simulink model "UnitTest_relay_model"  (Simulink 8.1)
settings: Solver=ode1  StartTime=0.0  StopTime=inf  FixedStep=Ts  MaxStep=1e-3  RelTol=1e-3
model workspace (MAT data in the model file):
  op_snapshot1 : opcond.OperatingPoint (value not decoded)
PostLoadFcn:
  | UnitTest_relay_model_init;
InitFcn:
  | UnitTest_relay_model_init;
values from neighbouring files (symbols this model uses):
  relay_par = xlsread('relay_parameters.xlsx')    [relay_settings_init.m]
  Ts = 100E-6    (= 0.0001)    [UnitTest_relay_model_init.m]
undefined symbols (not defined in the file or in its folder): cable_spec
libraries: powerlib x2, artemis x1, rtlab x1, breaker_lib x1, Load_lib x1, relay_modbus_lib x1, rtio_generic_modbus x1, cables_lib x1, transformer_lib x1
settings Model: ARTEMISmethode_block_infos=$$__separator__$$UnitTest_relay_model/ARTEMIS Guide$$__separator__$$  Creator=RE25624  LastModifiedBy=re25624  BufferReuse=off
settings SolverCC: ZeroCrossAlgorithm=Adaptive
settings DataIOCC: ExternalInput=getinputstruct(op_snapshot1)  InitialState=getstatestruct(op_snapshot1)  LimitDataPoints=off  MaxDataPoints=90060  SignalLoggingSaveFormat=Dataset  SaveOutput=off  SignalLogging=off  DSMLogging=off  SaveTime=off  OutputSaveName=result
settings OptimizationCC: BlockReduction=off  OptimizeBlockIOStorage=off  BufferReuse=off  ExpressionFolding=off  LocalBlockOutputs=off
settings DebuggingCC: MaxConsecutiveZCsMsg=warning  IgnoredZcDiagnostic=none  SolverPrmCheckMsg=none  MultiTaskRateTransMsg=warning  FcnCallInpInsideContextMsg=EnableAllAsWarning  FrameProcessingCompatibilityMsg=error  ModelReferenceExtraNoncontSigs=warning  StrictBusMsg=None
settings ModelReferenceCC: UpdateModelReferenceTargets=IfOutOfDate
settings SFSimCC: SFSimEcho=off
settings GRTTargetCC: CodeReplacementLibrary=C89/C90 (ANSI)

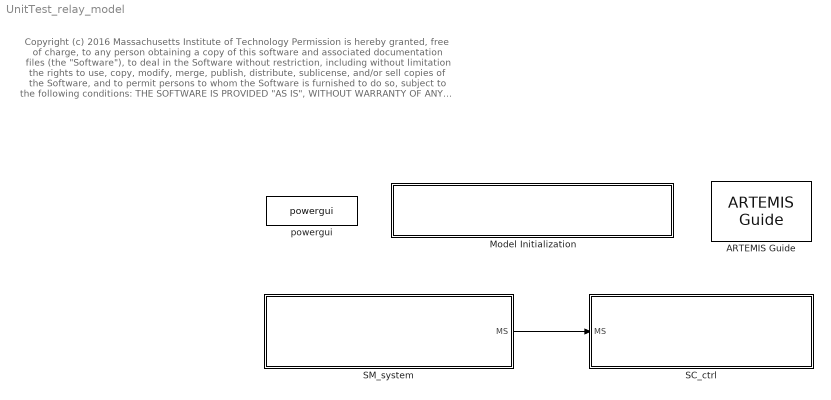
== system UnitTest_relay_model ==
  note: Copyright (c) 2016 Massachusetts Institute of Technology
      | Permission is hereby granted, free of charge, to any person obtaining a copy of this software and associated documentation files (the "Software"), to deal
      | in the Software without restriction, including without limitation the rights to use, copy, modify, merge, publish, distribute, sublicense, and/or sell copies of the
      | Software, and to permit persons to whom the Software is furnished to do so, subject to the following conditions:
      |
      | THE SOFTWARE IS PROVIDED "AS IS", WITHOUT WARRANTY OF ANY KIND, EXPRESS OR IMPLIED, INCLUDING BUT NOT LIMITED TO THE
      | WARRANTIES OF MERCHANTABILITY, FITNESS FOR A PARTICULAR PURPOSE AND NONINFRINGEMENT. IN NO EVENT SHALL THE AUTHORS
      | OR COPYRIGHT HOLDERS BE LIABLE FOR ANY CLAIM, DAMAGES OR OTHER LIABILITY, WHETHER IN AN ACTION OF CONTRACT, TORT OR
      | OTHERWISE, ARISING FROM, OUT OF OR IN CONNECTION WITH THE SOFTWARE OR THE USE OR OTHER DEALINGS IN THE SOFTWARE.
  ARTEMIS Guide : artemis/ARTEMIS/ARTEMIS Guide  Tag=FTSSmethode_opal_4hx0r99  Description=5.0_z1  lock=on  Ts=Ts  opt=art5  dyna=off  nb_perm=4  RT_fullcomp=off  ssn=on  ssn_itvc=off  ssn_ivic=off  ssn_ext=off  ssn_solver=Art5 with Backward Euler nodal interface  ssn_impulse=off  ssn_quasimpulse=off  ssn_impulse_loop=2  paraExtinctionThy=off  Thy_Impulse=on  dtc=Off  dtc_opt=normal  ao=on  simtype=off  ct_mac=off  lin_mov=off  lsp=[0.001 2]  spike_skip=Disabled  dtc_extra=1  dtc_sws=normal  dtc_pied=0.5  SPSRulesBlock=SPSRules  tre=on  ctmm=off  LF=off  dpl_type=ARTEMiS DPL  rlc_type=off  custom_type=off  para=on  ssn_ImpulseLoopBlockedStateUpdate=2  ssn_mov_iter_number=5  ssn_switch_iter_number=5
  Model Initialization : Subsystem  AncestorBlock=artemis/Tools /Misc/Model Initialization  mask(Model Functions){InitFcnX=UnitTest_relay_model_init;, prel=off, posl=on, inif=on, strf=off}
      mask prompts: InitFcnX "Initialisation"; prel "Preload Function"; posl "PostLoad Function"; inif "InitFcn"; strf "StartFcn"
      mask init:
      | currentBlock = gcb;
      | root = bdroot(currentBlock);
      | 
      | 
      | if ~strcmp(get_param(root,'BlockDiagramType'),'library')
      |     if prel==1
      |         set_param(root, 'PreLoadFcn', InitFcnX);
      |     else
      |         set_param(root, 'PreLoadFcn', '');
      |     end
      |     if inif==1
      |         set_param(root, 'InitFcn', InitFcnX);
      |     else
      |         set_param(root, 'InitFcn', '');
      |     end
      |     if strf==1
      |         set_param(root, 'StartFcn', InitFcnX);
      |     else
      |         set_param(root, 'StartFcn', '');
      |     end
      |     if posl==1
      |         set_param(root, 'PostLoadFcn', InitFcnX);
      |     else
      |         set_param(root, 'PostLoadFcn', '');
      |     end
      | end
      | 
      | pos = get_param(currentBlock, 'Position');
      | width = pos(3) - pos(1); height = pos(4) - pos(2);
      | txt = [ upper(root) '\n' '- InitFcn. . . . . '  get_param(root, 'InitFcn') ];
      settings: CopyFcn=set_param(gcb,'LinkStatus','inactive')
      mask Display: text(5, height*0.5, txt, 'horizontalAlignment', 'left', 'verticalAlignment', 'middle') ;
  SC_ctrl : Subsystem
  SM_system : Subsystem
  powergui : powerlib/powergui  Priority=2  SimulationMode=Discrete  SolverType=Tustin  SampleTime=Ts  frequency=60  SPID=off  DisableSnubberDevices=off  DisableRonSwitches=off  DisableVfSwitches=off  SwTol=0  Interpol=off  DisplayEquations=off  frequencyindice=0  Pbase=100e6  ErrMax=1e-4  Iterations=50  UnitsV=kV  UnitsW=MW  FunctionMessages=off  echomessages=off  HookPort=off  EnableUseOfTLC=off  x0status=blocks  RestoreLinks=warning  ResistiveCurrentMeasurement=off  Frange=logspace(0,3,50)  Ylog=off  Xlog=off  ShowGrid=off  save=off  variable=ZData  structure=0  ZoomFFT=on  StartTime=0.0  cycles=2  DisplayStyle=off  fundamental=60  FreqAxis=off  MaxFrequency=1000  frequencyindicesteady=1  RmsSteady=1  display=off  Ts=0  methode=off
  wires:
  SM_system/1(MS) -> SC_ctrl/1(MS)

== system UnitTest_relay_model/Model Initialization ==

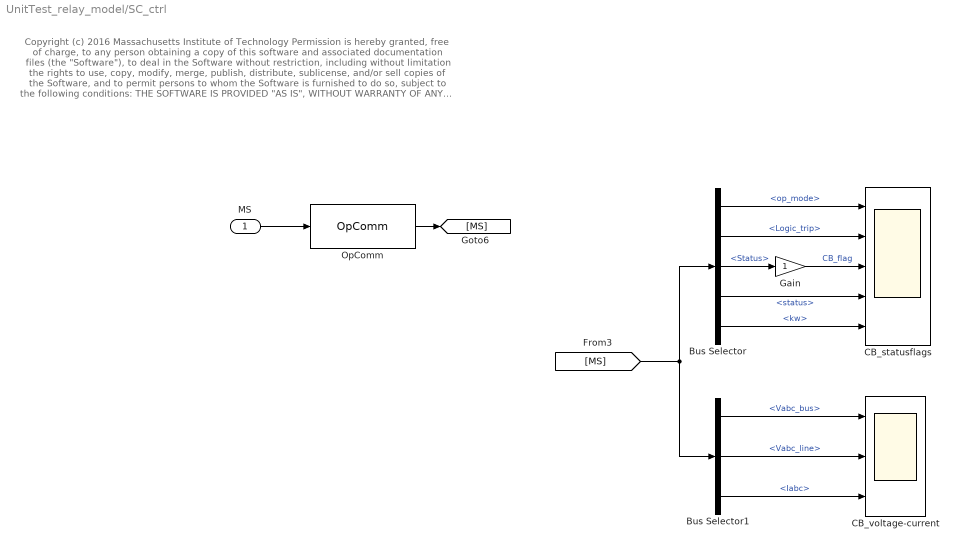
== system UnitTest_relay_model/SC_ctrl ==
  note: Copyright (c) 2016 Massachusetts Institute of Technology
      | Permission is hereby granted, free of charge, to any person obtaining a copy of this software and associated documentation files (the "Software"), to deal
      | in the Software without restriction, including without limitation the rights to use, copy, modify, merge, publish, distribute, sublicense, and/or sell copies of the
      | Software, and to permit persons to whom the Software is furnished to do so, subject to the following conditions:
      |
      | THE SOFTWARE IS PROVIDED "AS IS", WITHOUT WARRANTY OF ANY KIND, EXPRESS OR IMPLIED, INCLUDING BUT NOT LIMITED TO THE
      | WARRANTIES OF MERCHANTABILITY, FITNESS FOR A PARTICULAR PURPOSE AND NONINFRINGEMENT. IN NO EVENT SHALL THE AUTHORS
      | OR COPYRIGHT HOLDERS BE LIABLE FOR ANY CLAIM, DAMAGES OR OTHER LIABILITY, WHETHER IN AN ACTION OF CONTRACT, TORT OR
      | OTHERWISE, ARISING FROM, OUT OF OR IN CONNECTION WITH THE SOFTWARE OR THE USE OR OTHER DEALINGS IN THE SOFTWARE
  MS : Inport
  Bus Selector : BusSelector  OutputSignals=relay_cmd.op_mode,relay_cmd.Logic_trip,CB.Status,relay_cmd.m.status,relay_cmd.m.kw
  Bus Selector1 : BusSelector  OutputSignals=CB.Vabc_bus,CB.Vabc_line,CB.Iabc
  CB_statusflags : Scope  NumInputPorts=5
      settings: ShowLegends=on  TimeRange=16  YMin=-1~0~0~0~0  YMax=1~1~1~3~2000  SaveName=ScopeData6
  CB_voltage-current : Scope  NumInputPorts=3
      settings: ShowLegends=on  TimeRange=16  YMin=-15000~-15000~-150  YMax=15000~15000~150
  Gain : Gain
  OpComm : rtlab/OpComm  nbport=1  groupe_acq=1  subsys_rate=0  st=0  Synchronization=on  Interpolation=on  Threshold=1.0  Missed_Data=off  Sim_Time=off  Samples=off  dynSigOut=off  from_console=0  warning_done=off  writeOpCommFile=off  Offset=off
  wires:
  OpComm/1 -> [MS]
  MS/1 -> OpComm/1
  [MS] -> Bus Selector/1, Bus Selector1/1
  Bus Selector/5 -> CB_statusflags/5  "<kw>"
  Bus Selector/1 -> CB_statusflags/1  "<op_mode>"
  Bus Selector/2 -> CB_statusflags/2  "<Logic_trip>"
  Bus Selector/4 -> CB_statusflags/4  "<status>"
  Bus Selector/3 -> Gain/1  "<Status>"
  Gain/1 -> CB_statusflags/3  "CB_flag"
  Bus Selector1/2 -> CB_voltage-current/2  "<Vabc_line>"
  Bus Selector1/1 -> CB_voltage-current/1  "<Vabc_bus>"
  Bus Selector1/3 -> CB_voltage-current/3  "<Iabc>"

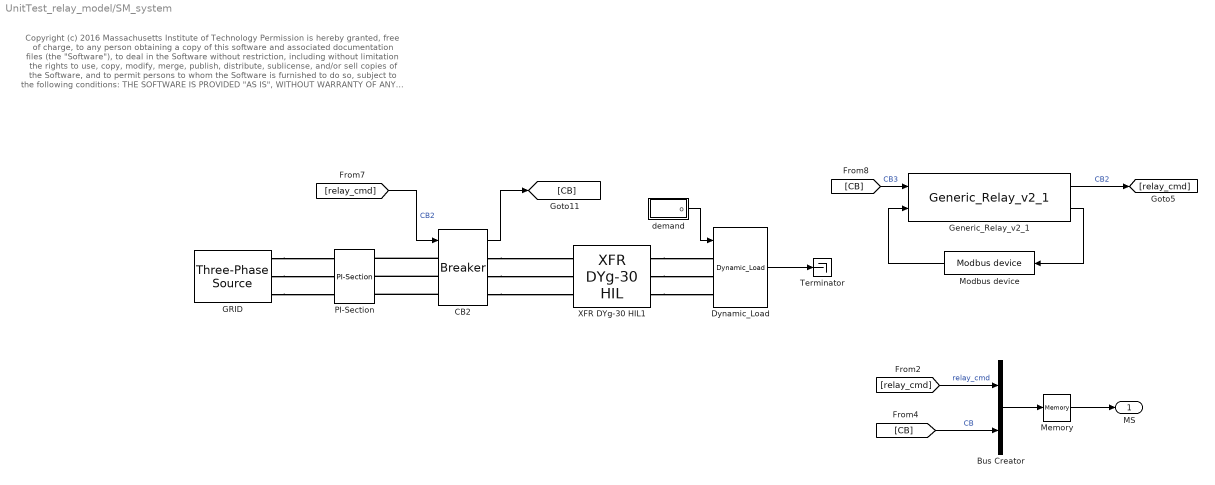
== system UnitTest_relay_model/SM_system ==
  note: Copyright (c) 2016 Massachusetts Institute of Technology
      | Permission is hereby granted, free of charge, to any person obtaining a copy of this software and associated documentation files (the "Software"), to deal
      | in the Software without restriction, including without limitation the rights to use, copy, modify, merge, publish, distribute, sublicense, and/or sell copies of the
      | Software, and to permit persons to whom the Software is furnished to do so, subject to the following conditions:
      |
      | THE SOFTWARE IS PROVIDED "AS IS", WITHOUT WARRANTY OF ANY KIND, EXPRESS OR IMPLIED, INCLUDING BUT NOT LIMITED TO THE
      | WARRANTIES OF MERCHANTABILITY, FITNESS FOR A PARTICULAR PURPOSE AND NONINFRINGEMENT. IN NO EVENT SHALL THE AUTHORS
      | OR COPYRIGHT HOLDERS BE LIABLE FOR ANY CLAIM, DAMAGES OR OTHER LIABILITY, WHETHER IN AN ACTION OF CONTRACT, TORT OR
      | OTHERWISE, ARISING FROM, OUT OF OR IN CONNECTION WITH THE SOFTWARE OR THE USE OR OTHER DEALINGS IN THE SOFTWARE
  Bus Creator : BusCreator  Inputs=2
  CB2 : breaker_lib/Breaker  Ts=Ts  mech_delay=cb_mech_delay
  Dynamic_Load : Load_lib/Dynamic_Load  V=480  Ts=Ts
  GRID : powerlib/Electrical Sources/Three-Phase Source  Voltage=13800  PhaseAngle=0  Frequency=60  InternalConnection=Yg  SpecifyImpedance=on  Resistance=0.8929  Inductance=16.58e-3  ShortCircuitLevel=375e6  BaseVoltage=13800  XRratio=30  BusType=swing  Pref=0  Qref=0  Qmin=-inf  Qmax=inf
  Generic_Relay_v2_1 : relay_modbus_lib/Generic_Relay_v2_1  Ts=Ts  relay_settings=[relay_par(2,:)]
  Memory : Memory
  Modbus device : rtio_generic_modbus/Modbus device  conf_name=F1_relay_cfg2.opal  conf_name_mask=F1_relay_cfg2.xls  sample_time=Ts
  PI-Section : cables_lib/PI-Section  cable_spec=[cable_spec(13, :)]  line_length=10000  parallel_sets=1
  Terminator : Terminator
  XFR DYg-30 HIL1 : transformer_lib/XFR DYg-30 HIL  Rating=2500  Vp=13800  Vs=480  Z=5.75  XR=6.6
  demand : Subsystem
  MS : Outport
  wires:
  CB2/1 -> [CB]
  Bus Creator/1 -> Memory/1
  [relay_cmd] -> Bus Creator/1  "relay_cmd"
  [CB] -> Bus Creator/2  "CB"
  Memory/1 -> MS/1
  Generic_Relay_v2_1/2 -> Modbus device/1
  [CB] -> Generic_Relay_v2_1/1  "CB3"
  Generic_Relay_v2_1/1 -> [relay_cmd]  "CB2"
  [relay_cmd] -> CB2/1  "CB2"
  Modbus device/1 -> Generic_Relay_v2_1/2
  demand/1(o) -> Dynamic_Load/1
  Dynamic_Load/1 -> Terminator/1
  connections:
  GRID/RConn3 -- PI-Section/LConn3
  GRID/RConn2 -- PI-Section/LConn2
  GRID/RConn1 -- PI-Section/LConn1
  CB2/LConn2 -- PI-Section/RConn2
  CB2/LConn1 -- PI-Section/RConn1
  CB2/LConn3 -- PI-Section/RConn3
  CB2/RConn1 -- XFR DYg-30 HIL1/LConn1
  CB2/RConn2 -- XFR DYg-30 HIL1/LConn2
  CB2/RConn3 -- XFR DYg-30 HIL1/LConn3
  XFR DYg-30 HIL1/RConn1 -- Dynamic_Load/LConn1
  XFR DYg-30 HIL1/RConn2 -- Dynamic_Load/LConn2
  XFR DYg-30 HIL1/RConn3 -- Dynamic_Load/LConn3

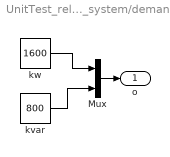
== system UnitTest_relay_model/SM_system/demand ==
  Mux : Mux  Inputs=2
  kvar : Constant  Value=800
  kw : Constant  Value=1600
  o : Outport
  wires:
  kw/1 -> Mux/1
  kvar/1 -> Mux/2
  Mux/1 -> o/1
